simulink model "DoorControlSystem"  (R2018a)
settings: Solver=FixedStepAuto  StartTime=0.0  StopTime=10.0  RelTol=1e-3  EnableMultiTasking=on
libraries: simulink x4
settings Model: ExtModeTrigDuration=2  Creator=fabricek  LastModifiedBy=fabricek
settings OptimizationCC: EnhancedBackFolding=on  PassReuseOutputArgsThreshold=0  MaxStackSize=64  OptimizeBlockOrder=speed  DifferentSizesBufferReuse=on  OptimizationCustomize=off
settings DebuggingCC: ParameterTunabilityLossMsg=error
settings HardwareCC: ProdBitPerInt=16  ProdBitPerPointer=16  ProdBitPerSizeT=16  ProdBitPerPtrDiffT=16  ProdLargestAtomicFloat=None  ProdWordSize=8  ProdHWDeviceType=Atmel->AVR  UseEmbeddedCoderFeatures=off  UseSimulinkCoderFeatures=off
settings SFSimCC: MATLABDynamicMemAlloc=off
settings RTWCC: SystemTargetFile=ert.tlc  HardwareBoard=Arduino Uno  TLCOptions=-aInlineSetEventsForThisBaseRateFcn=TLC_FALSE -aSuppressMultiTaskScheduler=TLC_FALSE -aRateBasedStepFcn=1  TemplateMakefile=ert_default_tmf  GenerateReport=on  Toolchain=Arduino AVR  BuildConfiguration=Faster Runs  LaunchReport=on
settings CodeAppCC: ForceParamTrailComments=on  OperatorAnnotations=on
settings ERTTargetCC: ERTCustomFileBanners=off  SupportContinuousTime=on  SupportNonInlinedSFcns=on  RemoveResetFunc=off  SupportVariableSizeSignals=on  ModelStepFunctionPrototypeControlCompliant=off

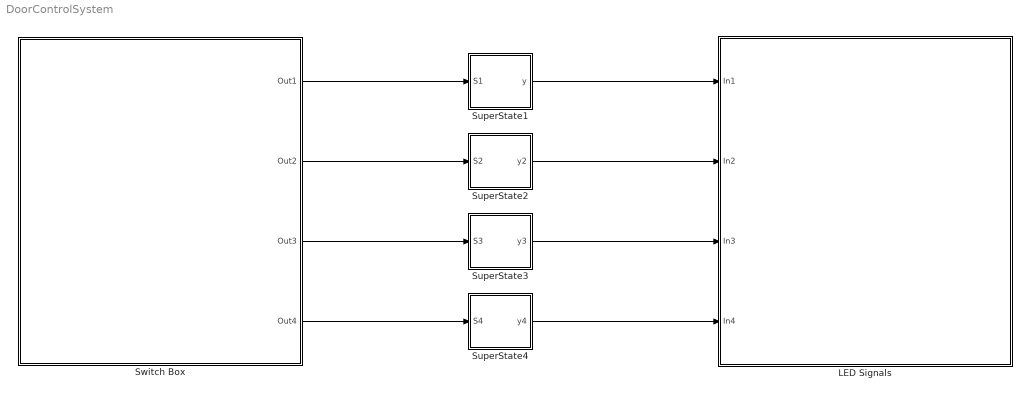
== system DoorControlSystem ==
  LED Signals : Subsystem
  SuperState1 : Stateflow chart  TreatAsAtomicUnit=on
  SuperState2 : Stateflow chart  TreatAsAtomicUnit=on
  SuperState3 : Stateflow chart  TreatAsAtomicUnit=on
  SuperState4 : Stateflow chart  TreatAsAtomicUnit=on
  Switch Box : Subsystem
  wires:
  SuperState3/1(y3) -> LED Signals/3(In3)
  SuperState2/1(y2) -> LED Signals/2(In2)
  Switch Box/3(Out3) -> SuperState3/1(S3)
  Switch Box/1(Out1) -> SuperState1/1(S1)
  SuperState1/1(y) -> LED Signals/1(In1)
  Switch Box/4(Out4) -> SuperState4/1(S4)
  SuperState4/1(y4) -> LED Signals/4(In4)
  Switch Box/2(Out2) -> SuperState2/1(S2)

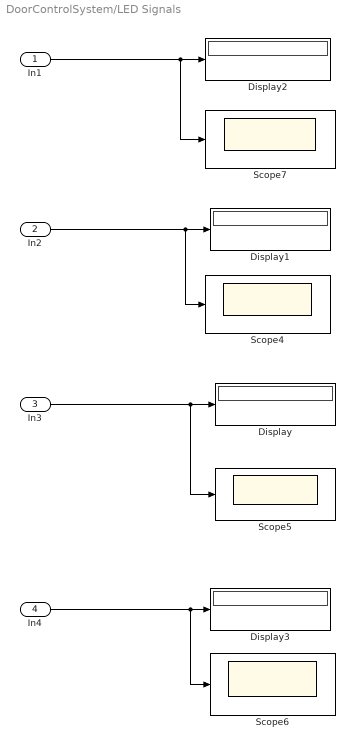
== system DoorControlSystem/LED Signals ==
  In1 : Inport
  In2 : Inport  Port=2
  In3 : Inport  Port=3
  In4 : Inport  Port=4
  Display{,1..3} (4 alike) : Display
  Scope{4..7} (4 alike) : Scope
  wires:
  In4/1 -> Display3/1, Scope6/1
  In1/1 -> Display2/1, Scope7/1
  In3/1 -> Scope5/1, Display/1
  In2/1 -> Display1/1, Scope4/1

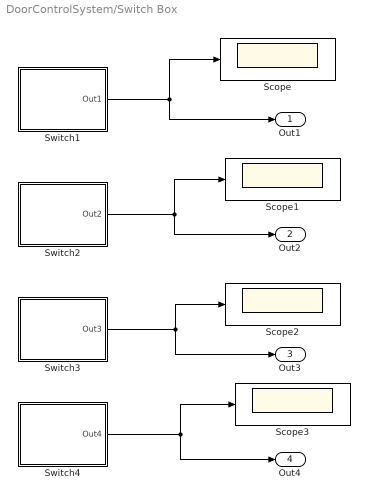
== system DoorControlSystem/Switch Box ==
  Scope{,1..3} (4 alike) : Scope
  Switch1 : Subsystem
  Switch2 : Subsystem
  Switch3 : Subsystem
  Switch4 : Subsystem
  Out1 : Outport
  Out2 : Outport  Port=2
  Out3 : Outport  Port=3
  Out4 : Outport  Port=4
  wires:
  Switch2/1(Out2) -> Out2/1, Scope1/1
  Switch3/1(Out3) -> Out3/1, Scope2/1
  Switch1/1(Out1) -> Out1/1, Scope/1
  Switch4/1(Out4) -> Out4/1, Scope3/1

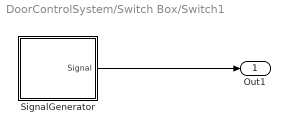
== system DoorControlSystem/Switch Box/Switch1 ==
  SignalGenerator : Subsystem
  Out1 : Outport
  wires:
  SignalGenerator/1(Signal) -> Out1/1

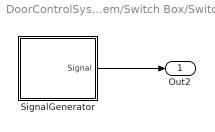
== system DoorControlSystem/Switch Box/Switch2 ==
  SignalGenerator : Subsystem
  Out2 : Outport
  wires:
  SignalGenerator/1(Signal) -> Out2/1

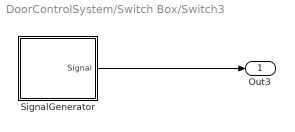
== system DoorControlSystem/Switch Box/Switch3 ==
  SignalGenerator : Subsystem
  Out3 : Outport
  wires:
  SignalGenerator/1(Signal) -> Out3/1

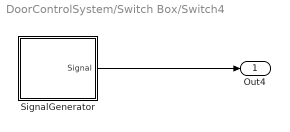
== system DoorControlSystem/Switch Box/Switch4 ==
  SignalGenerator : Subsystem
  Out4 : Outport
  wires:
  SignalGenerator/1(Signal) -> Out4/1

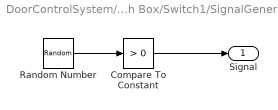
== system DoorControlSystem/Switch Box/Switch1/SignalGenerator ==
  Compare To Constant : simulink/Logic and Bit Operations/Compare To Constant  relop=>  const=0  OutDataTypeStr=boolean
  Random Number : RandomNumber  Mean=1  SampleTime=0.1
  Signal : Outport
  wires:
  Compare To Constant/1 -> Signal/1
  Random Number/1 -> Compare To Constant/1

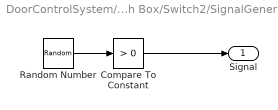
== system DoorControlSystem/Switch Box/Switch2/SignalGenerator ==
  Compare To Constant : simulink/Logic and Bit Operations/Compare To Constant  relop=>  const=0  OutDataTypeStr=boolean
  Random Number : RandomNumber  Mean=1  SampleTime=0.1
  Signal : Outport
  wires:
  Compare To Constant/1 -> Signal/1
  Random Number/1 -> Compare To Constant/1

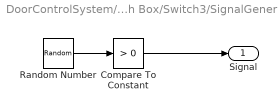
== system DoorControlSystem/Switch Box/Switch3/SignalGenerator ==
  Compare To Constant : simulink/Logic and Bit Operations/Compare To Constant  relop=>  const=0  OutDataTypeStr=boolean
  Random Number : RandomNumber  Mean=1  SampleTime=0.1
  Signal : Outport
  wires:
  Compare To Constant/1 -> Signal/1
  Random Number/1 -> Compare To Constant/1

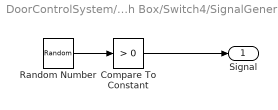
== system DoorControlSystem/Switch Box/Switch4/SignalGenerator ==
  Compare To Constant : simulink/Logic and Bit Operations/Compare To Constant  relop=>  const=0  OutDataTypeStr=boolean
  Random Number : RandomNumber  Mean=1  SampleTime=0.1
  Signal : Outport
  wires:
  Compare To Constant/1 -> Signal/1
  Random Number/1 -> Compare To Constant/1

== stateflow chart DoorControlSystem/SuperState2 ==
  state IdleState
  state LED2_ON
    entry:
    y2 = 1;
  state LED2_OFF
    entry:
    y2 = 0;
  (default) -> IdleState
  LED2_ON -> IdleState
  IdleState -> LED2_ON [order 2] : [S2 == 1]
  LED2_OFF -> IdleState
  IdleState -> LED2_OFF [order 1] : [S2 == 0]
  data: y2 output; S2 input

== stateflow chart DoorControlSystem/SuperState4 ==
  state IdleState
  state LED4_ON
    entry:
    y4 = 1;
  state LED4_OFF
    entry:
    y4 = 0;
  (default) -> IdleState
  IdleState -> LED4_ON [order 1] : [S4 == 1]
  LED4_ON -> IdleState
  LED4_OFF -> IdleState
  IdleState -> LED4_OFF [order 2] : [S4 == 0]
  data: y4 output; S4 input

== stateflow chart DoorControlSystem/SuperState1 ==
  state IdleState
  state LED1_ON
    entry:y =1;
  state LED1_OFF
    entry:
    y=0;
  (default) -> IdleState
  IdleState -> LED1_ON [order 1] : [S1 == 1]
  LED1_ON -> IdleState
  LED1_OFF -> IdleState
  IdleState -> LED1_OFF [order 2] : [S1 == 0]
  data: y output; S1 input

== stateflow chart DoorControlSystem/SuperState3 ==
  state LED3_ON
    entry:
    y3 = 1;
  state IdleState
  state LED3_OFF
    entry:
    y3 = 0;
  IdleState -> LED3_ON [order 1] : [S3 == 1]
  (default) -> IdleState
  LED3_ON -> IdleState
  LED3_OFF -> IdleState
  IdleState -> LED3_OFF [order 2] : [S3 == 0]
  data: y3 output; S3 input
